simulink model "FTS_Spiral_June18"  (R2018a)
settings: Solver=FixedStepDiscrete  StartTime=0.0  StopTime=5  FixedStep=0.01  RelTol=1e-3  EnableMultiTasking=on
settings Model: Creator=rhamrah  LastModifiedBy=akrobotix
settings OptimizationCC: LifeSpan=inf
settings DebuggingCC: SFUnexpectedBacktrackingDiag=warning  SFNoUnconditionalDefaultTransitionDiag=warning  SFExecutionAtInitializationDiag=none
settings CodeAppCC: StateflowObjectComments=on
settings GRTTargetCC: TargetLangStandard=C89/C90 (ANSI)  GeneratePreprocessorConditionals=Disable all
settings ConfigComp: CovMetricSettings=dw  CovHtmlReporting=on  CovSaveCumulativeToWorkspaceVar=on  CovSaveSingleToWorkspaceVar=on  CovExternalEMLEnable=off

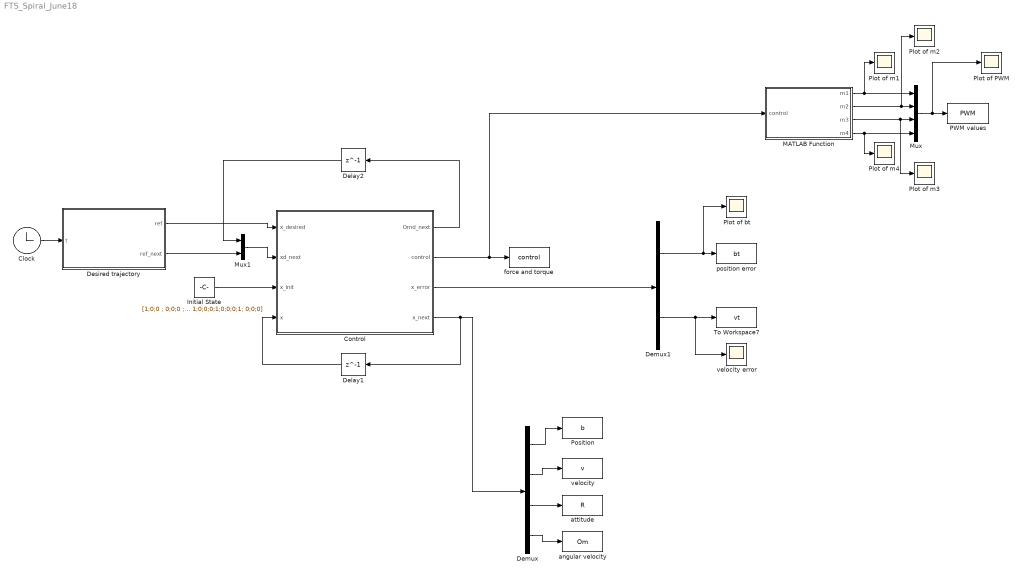
== system FTS_Spiral_June18 ==
  Clock : Clock
  Control : MATLAB Function  TreatAsAtomicUnit=on
  Delay1 : Delay  DelayLength=1  InitialCondition=0
  Delay2 : Delay  DelayLength=1  InitialCondition=0
  Demux : Demux  Outputs=[3 3 9 3]
  Demux1 : Demux  Outputs=[3 3]
  Desired trajectory : MATLAB Function  TreatAsAtomicUnit=on
  Initial State : Constant  Value=[1;0;0 ; 0;0;0 ; 1;0;0;0;1;0;0;0;1; 0;0;0]
  MATLAB Function : MATLAB Function  TreatAsAtomicUnit=on
  Mux : Mux
  Mux1 : Mux  Inputs=2
  PWM values : ToWorkspace  VariableName=PWM  SaveFormat=Timeseries  SampleTime=-1
  Plot of PWM : Scope
  Plot of bt : Scope
  Plot of m{1..4} (4 alike) : Scope
  Position : ToWorkspace  VariableName=b  SaveFormat=Structure  SampleTime=-1
  To Workspace7 : ToWorkspace  VariableName=vt  SaveFormat=Structure  SampleTime=-1
  angular velocity : ToWorkspace  VariableName=Om  SaveFormat=Structure  SampleTime=-1
  attitude : ToWorkspace  VariableName=R  SaveFormat=Structure  SampleTime=-1
  force and torque : ToWorkspace  VariableName=control  SaveFormat=Structure  SampleTime=-1
  position error : ToWorkspace  VariableName=bt  SaveFormat=Structure  SampleTime=-1
  velocity : ToWorkspace  VariableName=v  SaveFormat=Structure  SampleTime=-1
  velocity error : Scope
  wires:
  Desired trajectory/1(ref) -> Control/1(x_desired)
  Clock/1 -> Desired trajectory/1("t ")
  Delay1/1 -> Control/4(x)
  Initial State/1 -> Control/3(x_init)
  Control/4(x_next) -> Demux/1, Delay1/1
  Control/1(Omd_next) -> Delay2/1
  Mux1/1 -> Control/2(xd_next)
  Delay2/1 -> Mux1/1
  Demux/2 -> velocity/1
  Demux/1 -> Position/1
  Desired trajectory/2(ref_next) -> Mux1/2
  Demux/3 -> attitude/1
  Demux/4 -> angular velocity/1
  Control/3(x_error) -> Demux1/1
  Demux1/2 -> To Workspace7/1, velocity error/1
  Demux1/1 -> Plot of bt/1, position error/1
  Mux/1 -> Plot of PWM/1, PWM values/1
  MATLAB Function/1(m1) -> Plot of m1/1, Mux/1
  Control/2(control) -> MATLAB Function/1(control), force and torque/1
  MATLAB Function/4(m4) -> Plot of m4/1, Mux/4
  MATLAB Function/3(m3) -> Plot of m3/1, Mux/3
  MATLAB Function/2(m2) -> Plot of m2/1, Mux/2

== matlab function FTS_Spiral_June18/Desired trajectory ==
  data: t input size=1; ref output size=[10 1]; ref_next output size=[9 1]
% desired traj

function [ref,ref_next] = desired_traj(t)

h=0.01;

% t(k+1) = t+h;

bd = [0.4*sin(pi*t);0.6*cos(pi*t);0.4*t];
vd = [0.4*pi*cos(pi*t);-0.6*pi*sin(pi*t);0.4];
dvd = [-0.4*pi^2*sin(pi*t);-0.6*pi^2*cos(pi*t);0];

ref = [bd;vd;dvd;t];


bd_next = [0.4*sin(pi*(t+h));0.6*cos(pi*(t+h));0.4*(t+h)];
vd_next = [0.4*pi*cos(pi*(t+h));-0.6*pi*sin(pi*(t+h));0.4];
dvd_next = [-0.4*pi^2*sin(pi*(t+h));-0.6*pi^2*cos(pi*(t+h));0];

ref_next = [bd_next;vd_next;dvd_next];
end

== matlab function FTS_Spiral_June18/Control ==
  data: Omd_next output size=[3 1]; control output size=[4 1]; x_error output size=[6 1]; x_next output size=[18 1]; x_desired input; xd_next input; x_init input; x input
function [Omd_next,control,x_error,x_next]  = newFTS(x_desired,xd_next,x_init,x)

J=diag([0.0820,0.0845,0.1377]);         % kgm^2
m=4.34;                                 % kg
M=m*eye(3);
g=9.81;
h = 0.01;
e3=[0;0;1];


% x_next = zeros(18,1);

t = x_desired(10);

if t==0
b = x_init(1:3,:);
nu = x_init(4:6,:);
R = reshape(x_init(7:15,:),3,3);
Om = x_init(16:18,:);
Omd = Om;
% 
% bd = x_desired(1:3,:);
% vd = x_desired(4:6,:);
% dvd = x_desired(7:9,:);
% 
% bt = b - bd;
% vt = R*nu - vd;
% Rd = desired_attitude(bt,vt,dvd);

else
    b = x(1:3,:);
    nu = x(4:6,:);
    R = reshape(x(7:15,:),3,3);
    Om = x(16:18,:);
    
%     bd = x_desired(1:3,:);
%     vd = x_desired(4:6,:);
%     dvd = x_desired(7:9,:);
% 
%     bt = xt(1:3,:);
%     vt = xt(4:6,:);
%     Rd = desired_attitude(bt,vt,dvd);
    
    Omd = xd_next(1:3,:);
end

bd = x_desired(1:3,:);
vd = x_desired(4:6,:);
dvd = x_desired(7:9,:);

bd_next = xd_next(4:6,:);
vd_next = xd_next(7:9,:);
dvd_next = xd_next(10:12,:);

bt = b - bd;
vt = R*nu - vd;
Rd = desired_attitude(bt,vt,dvd);


fi = h*Om;
F = expmso3(fi);
    
R_next = R*F;       % next attitude
b_next = h*R*nu + b; % the next position

bt_next = b_next - bd_next;

% The control torque:
fm = trans_control_f(R,bt,nu,vd,dvd);

nu_next = M\(F'*M*nu + h*m*g*R_next'*e3 - h*fm*e3);
v_next = R_next*nu_next;

vt_next = v_next - vd_next;
    
Rd_next = desired_attitude(bt_next,vt_next,dvd_next);
    
Fd_next = Rd'*Rd_next;
    
Omd_next = (1/h)*(logmso3(Fd_next));
    
dOmd = (1/h)*(Omd_next - Omd);
    
Q = Rd'*R;
    
%om(:,k)=Om(:,k)-Q(:,:,k)'*Omd(:,k)
   
tau = attitude_control_tau(Om,Omd,dOmd,Q);
        
Om_next = J\((F'*J*Om)+ h*tau);

control = [fm ; tau];
x_next = [b_next;nu_next;reshape(R_next,9,1);Om_next];

x_error = [bt;vt];


% bd=[0.2*t;.5*t;0.04*t];
% vd=[0.2;0.5;.04];
% dvd=[0;0; 0];
% ----------------------------------
% J=[-0.71 0.71 0; -0.71 -0.71 0 ; 0 0 1] ;         % kgm^2
% m=.5;                                 % kg
% M=m*eye(3);
% g=9.81;
% h = 0.01;
% 
% e1=[1;0;0;];e2=[0;1;0];e3=[0;0;1];
% 
% P=.2*eye(3);
% L=.5*eye(3);
% 
% La=3*eye(3);
% p=11/9;
% ki =.05;%0.098;%3
% kp = .5;%>1

%VICON IN THE LOOP
% b = x(1:3);
% v = x(4:6);
% R = reshape(x(7:15,:),3,3);
% Om = x(16:18,:);
% t = x(19,:);
% 
% h = 0.01;
% bd = x_desired(1:3,:);
% vd = x_desired(4:6,:);
% dvd = x_desired(7:9,:);
% 
% bt = b - bd;
% vt = v - vd;
% Rd=desired_attitude(bt,vt,dvd);

% %     R(:,:,k+1)=R(:,:,k)*F(:,:,k);       % next attitude
% %     b(:,k+1)=h*R(:,:,k)*nu(:,k)+b(:,k); % the next position
% %     
% %     % The control torque:
% %     bt(:,k+1)=b(:,k+1)-bd(:,k+1);
%     
%     nu = inv(R)*v;
%     fm = trans_control_f(R,bt,nu,vd,dvd);
%     
%     Rd_past = reshape(past_desired(10:18),3,3);
%     
%     Fd = Rd_past'*Rd;
%     
%     Omd = (1/h)*(logmso3(Fd));
%     Omd_past = past_desired(18:21);
%     
%     dOmd=(1/h)*(Omd-Omd_past);
%     
%     Q = Rd'*R;
%     
%     %om(:,k)=Om(:,k)-Q(:,:,k)'*Omd(:,k)
%    
%     tau = attitude_control_tau(Om, Omd, dOmd , Q );
%         
%     Om = J\((F'*J*Om)+h*tau);
%     
%     control = [fm ; Om];
% ----------------------------------
    
end

== matlab function FTS_Spiral_June18/MATLAB Function ==
  data: control input; m1 output; m2 output; m3 output; m4 output
% mapping
function [m1, m2, m3, m4] = PWMmap(control)

f = control(1,:);
tau = control (2:4,:);

 
 p1 =  0.00751;  %0.009334;
% sum of the constant terms 
 p2 =    -8.45436; % -9.711;
 
% diagonal distance in meters      
 D = sqrt(2)*0.14891;
  
% torque constant            
 p3 =  0.00011;  %0.0001189;
%p4 =     -0.112; 


K = [ 0 -p1*D 0 p1*D; p1*D 0 -p1*D 0; -p3 p3 -p3 p3; -p1 -p1 -p1 -p1];
%K^(-1);
% Kinv = (1/4)*[ 0 2/(p1*D) -1/p3 1/p1; -2/(p1*D) 0 1/p3 1/p1; 0 -2/(p1*D) -1/p3 1/p1;...
%             2/(p1*D) 0 1/p3 1/p1];

 %       -4*p2
        
%K*Kinv;
fmod = f-4*p2;

M = inv(K)*[tau(1); tau(2); tau(3); fmod]; 
m1 = M(1);
m2 = M(2);
m3 = M(3);
m4 = M(4);
       
end
